simulink model "TestSetpointTransitionHandler"  (R2016b)
settings: Solver=FixedStepAuto  StartTime=0.0  StopTime=20  FixedStep=0.002  RelTol=1e-3  EnableMultiTasking=on
undefined symbols (not defined in the file or in its folder): ControlStrategy
libraries: slrtlib x4, simulink x2
settings Model: SimulationMode=external  Creator=march  LastModifiedBy=march
settings SolverCC: EnableConcurrentExecution=on
settings DataIOCC: SaveFormat=StructureWithTime
settings OptimizationCC: BlockReduction=off  OptimizeBlockIOStorage=off  BufferReuse=off  GlobalBufferReuse=off  ExpressionFolding=off  LocalBlockOutputs=off
settings HardwareCC: ProdBitPerPointer=32  ProdBitPerSizeT=32  ProdBitPerPtrDiffT=32  ProdLargestAtomicFloat=None  ProdWordSize=32  ProdLongLongMode=on  ProdHWDeviceType=Generic->32-bit x86 compatible
settings RTWCC: SystemTargetFile=slrt.tlc  TemplateMakefile=slrt_default_tmf  Description=Simulink Real-Time  RTWCompilerOptimization=on

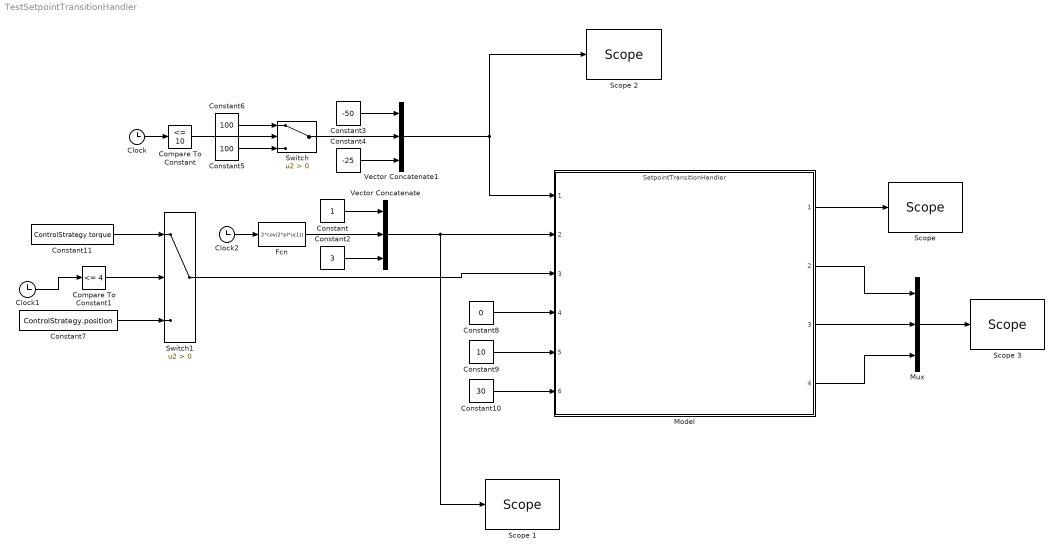
== system TestSetpointTransitionHandler ==
  Clock : Clock
  Clock1 : Clock
  Clock2 : Clock
  Compare To Constant : simulink/Logic and Bit Operations/Compare To Constant  relop=<=  const=10  OutDataTypeStr=boolean
  Compare To Constant1 : simulink/Logic and Bit Operations/Compare To Constant  relop=<=  const=4  OutDataTypeStr=boolean
  Constant : Constant
  Constant10 : Constant  Value=30
  Constant11 : Constant  Value=ControlStrategy.torque
  Constant2 : Constant  Value=3
  Constant3 : Constant  Value=-50
  Constant4 : Constant  Value=-25
  Constant5 : Constant  Value=100
  Constant6 : Constant  Value=100
  Constant7 : Constant  Value=ControlStrategy.position
  Constant8 : Constant  Value=0
  Constant9 : Constant  Value=10
  Fcn : Fcn  Expr=2*cos(2*pi*u(1))
  Model : ModelReference  ModelNameDialog=SetpointTransitionHandler  SimulationMode=Normal  ModelReferenceVersion=1.41
  Mux : Mux  Inputs=3
  "Scope " : slrtlib/Displays and Logging/Scope   scopeno=1  scopetype=Target  autostart=on  viewmode=Graphical rolling  formatstr='%15.6f'  grid=on  ylimits=[-100,100]  nosamples=250  noprepostsamples=0  interleave=1  triggermode=FreeRun  triggersignal=1  trigsignalfromport=off  triggerlevel=0.0  triggerslope=Either  triggerscope=1  triggersample=0  filename=data.dat  mode=Lazy  writesize=512  autorestart=off  dynamicfilemode=off  maxwritefilesize=512*1024^2
  Scope 1 : slrtlib/Displays and Logging/Scope   scopeno=2  scopetype=Target  autostart=on  viewmode=Graphical rolling  formatstr='%15.6f'  grid=on  ylimits=[-10,10]  nosamples=250  noprepostsamples=0  interleave=1  triggermode=FreeRun  triggersignal=1  trigsignalfromport=off  triggerlevel=0.0  triggerslope=Either  triggerscope=1  triggersample=0  filename=data.dat  mode=Lazy  writesize=512  autorestart=off  dynamicfilemode=off  maxwritefilesize=512*1024^2
  Scope 2 : slrtlib/Displays and Logging/Scope   scopeno=3  scopetype=Target  autostart=on  viewmode=Graphical rolling  formatstr='%15.6f'  grid=on  ylimits=[-150,150]  nosamples=250  noprepostsamples=0  interleave=1  triggermode=FreeRun  triggersignal=1  trigsignalfromport=off  triggerlevel=0.0  triggerslope=Either  triggerscope=1  triggersample=0  filename=data.dat  mode=Lazy  writesize=512  autorestart=off  dynamicfilemode=off  maxwritefilesize=512*1024^2
  Scope 3 : slrtlib/Displays and Logging/Scope   scopeno=4  scopetype=Target  autostart=on  viewmode=Numerical  formatstr='%15.6f'  grid=on  ylimits=[0,0]  nosamples=250  noprepostsamples=0  interleave=1  triggermode=FreeRun  triggersignal=1  trigsignalfromport=off  triggerlevel=0.0  triggerslope=Either  triggerscope=1  triggersample=0  filename=data.dat  mode=Lazy  writesize=512  autorestart=off  dynamicfilemode=off  maxwritefilesize=512*1024^2
  Switch : Switch  Criteria=u2 > Threshold
  Switch1 : Switch  Criteria=u2 > Threshold
  Vector Concatenate : Concatenate  NumInputs=3
  Vector Concatenate1 : Concatenate  NumInputs=3
  wires:
  Fcn/1 -> Vector Concatenate/2
  Constant/1 -> Vector Concatenate/1
  Constant2/1 -> Vector Concatenate/3
  Vector Concatenate/1 -> Scope 1/1, Model/2
  Clock/1 -> Compare To Constant/1
  Compare To Constant/1 -> Switch/2
  Constant5/1 -> Switch/3
  Constant6/1 -> Switch/1
  Vector Concatenate1/1 -> Scope 2/1, Model/1
  Constant4/1 -> Vector Concatenate1/3
  Constant8/1 -> Model/4
  Constant9/1 -> Model/5
  Constant10/1 -> Model/6
  Model/1 -> "Scope "/1
  Constant3/1 -> Vector Concatenate1/1
  Switch/1 -> Vector Concatenate1/2
  Clock1/1 -> Compare To Constant1/1
  Compare To Constant1/1 -> Switch1/2
  Constant11/1 -> Switch1/1
  Constant7/1 -> Switch1/3
  Switch1/1 -> Model/3
  Mux/1 -> Scope 3/1
  Model/3 -> Mux/2
  Model/2 -> Mux/1
  Model/4 -> Mux/3
  Clock2/1 -> Fcn/1
